simulink model "fsm_exercise"  (R2024b)
settings: Solver=VariableStepAuto  StartTime=0.0  StopTime=30  RelTol=1e-3
libraries: simulink x4
settings Model: Creator=rlaco  LastModifiedBy=rlaco

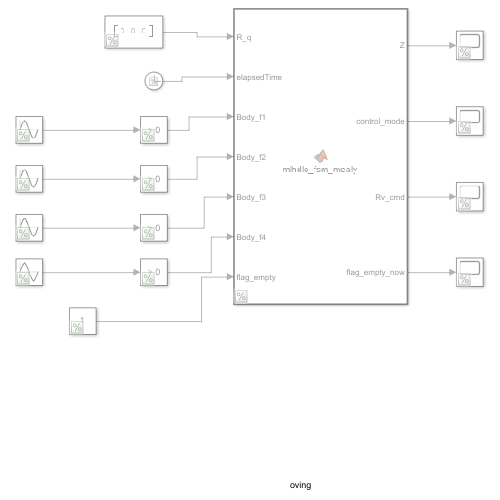
[thumbnail: Simulink's stored preview of the top-level diagram]
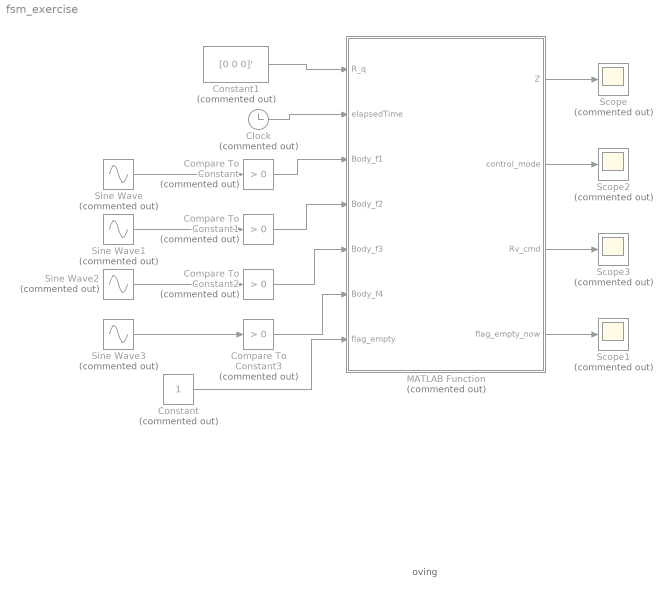
== system fsm_exercise ==
  note: oving
  Clock : Clock  Commented=on
  Compare To Constant{,1..3} (4 alike) : simulink/Logic and Bit Operations/Compare To Constant  Commented=on  relop=>  const=0  OutDataTypeStr=boolean
  Constant : Constant  Commented=on
  Constant1 : Constant  Commented=on  Value=[0 0 0]'
  MATLAB Function : MATLAB Function  Commented=on  TreatAsAtomicUnit=on
  Scope{,1..3} (4 alike) : Scope  Commented=on
  Sine Wave : Sin  Commented=on  SampleTime=0
  Sine Wave1 : Sin  Commented=on  Phase=60  SampleTime=0
  Sine Wave2 : Sin  Commented=on  Phase=90  SampleTime=0
  Sine Wave3 : Sin  Commented=on  Phase=100  SampleTime=0
  wires:
  Constant1/1 -> MATLAB Function/1(R_q)
  Clock/1 -> MATLAB Function/2(elapsedTime)
  MATLAB Function/1(Z) -> Scope/1
  Compare To Constant/1 -> MATLAB Function/3(Body_f1)
  Sine Wave/1 -> Compare To Constant/1
  MATLAB Function/2(control_mode) -> Scope2/1
  Sine Wave1/1 -> Compare To Constant1/1
  Sine Wave2/1 -> Compare To Constant2/1
  Sine Wave3/1 -> Compare To Constant3/1
  Compare To Constant1/1 -> MATLAB Function/4(Body_f2)
  Compare To Constant2/1 -> MATLAB Function/5(Body_f3)
  Compare To Constant3/1 -> MATLAB Function/6(Body_f4)
  MATLAB Function/4(flag_empty_now) -> Scope1/1
  MATLAB Function/3(Rv_cmd) -> Scope3/1
  Constant/1 -> MATLAB Function/7(flag_empty)

== matlab function fsm_exercise/MATLAB Function ==
  data: Z output; R_q input; elapsedTime input; Body_f1 input; control_mode output; Body_f2 input; Body_f3 input; Body_f4 input; Rv_cmd output; flag_empty input; flag_empty_now output
function [Z,control_mode,Rv_cmd,flag_empty_now]  = mlhdlc_fsm_mealy( R_q, elapsedTime, Body_f1, Body_f2, Body_f3, Body_f4, flag_empty)



% define states
S1 = 1; %% pre-grasping
S2 = 2; %% stay
S3 = 3; %% closing (grasping)
S4 = 4; %% touch
S5 = 5; %% empty

Rv_cmd = zeros(3,1); 
control_mode = zeros(3,1);
flag_empty_now =0;

persistent current_state

if isempty(current_state)
    current_state = S1;   
    current_state = 1;
end

Body_contact = (Body_f1 && Body_f2 && Body_f3 && Body_f4) || ...
               (Body_f1 && Body_f3) || (Body_f2 && Body_f4);

%% FSM start

if current_state == S1;
  
        
    R_condition_1 = (R_q(1) >= -45-2 && R_q(1) <= -45+2);
    R_condition_2 = (R_q(2) >= -5 && R_q(2) <= 5);
    R_condition_3 = (R_q(3) >= -5 && R_q(3) <= 5);
    
    R_condition = R_condition_1 && R_condition_2 && R_condition_3;

    % condition = R_condition;
    condition = 1;

    Rv_cmd = [-45 0 0]'*pi/180;
    control_mode = [1 1 1]';
    
    if (condition)
        if trackTime(elapsedTime, condition,1) >= 10
            current_state = 2;

            trackTime(elapsedTime, 0,1);
        end
    else
            current_state = 1;


    end
   
end

if current_state == S2


     if trackTime(elapsedTime, 1, 2) >= 10
        current_state = 3;
 
        durationTime_S2 = elapsedTime
        trackTime(elapsedTime, 0, 2);
     else
        current_state = 2;
        Rv_cmd = [0 0 0]'*pi/180;
        control_mode = [2 2 2]';

     end
end

if current_state == S3; %% closing

       Rv_cmd = [0.5 2 1.5]'*1*pi/180;
       control_mode = [2 2 2]';

    if flag_empty ==1
        Rv_cmd = [-0.5 -2 -1.5]'*1*pi/180;
       control_mode = [2 2 2]';

       flag_empty_now =1;
    else
       flag_empty_now =0;
    end 

    if Body_contact == 1
       grasped_time = trackTime(elapsedTime, 1,3);

        if grasped_time>=1
            current_state = 2;
            trackTime(elapsedTime, 0,3);
        end
    else
        trackTime(elapsedTime, 0,3);
    end
end

 Z = current_state

end



function [temp] = trackTime(elapsedTime, timer_flg, id)
    persistent isTiming startTime totalDuration
    temp = 0;

    if isempty(isTiming)
        isTiming = false(10,1);  % 최대 10개의 타이머 ID 지원
        startTime = zeros(10,1);
        totalDuration = zeros(10,1);
    end


    if timer_flg == 1 && ~isTiming(id)
        startTime(id) = elapsedTime;
        isTiming(id) = true;


    elseif timer_flg == 1 && isTiming(id)
        currentDuration = elapsedTime - startTime(id);
        temp = currentDuration;


    elseif timer_flg == 0 && isTiming(id)
        totalDuration(id) = elapsedTime - startTime(id);

        isTiming(id) = false;
        startTime(id) = 0;
        totalDuration(id) = 0;
    end
end
